simulink model "DAQ_DB_Test"  (Simulink 4.00)
settings: Solver=FixedStepDiscrete  StartTime=0.0  StopTime=inf  FixedStep=0.05  RelTol=1e-3
settings Model: LastModifiedBy=bsaunder

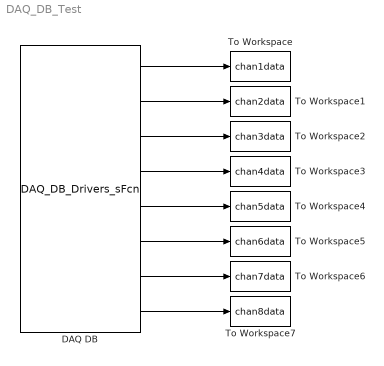
== system DAQ_DB_Test ==
  DAQ DB : S-Function  FunctionName=DAQ_DB_Drivers_sFcn  Parameters=Ts, (channels-1), gains, scanRate  PortCounts=[]  SFunctionModules=''  mask(DAQ_DB){channels=[1 2 3 4 5 6 7 8], gains=[1 1 1 1 1 1 1 1], scanRate=150, Ts=0.05}
      mask prompts: scanRate "Number of scans per sample time"; Ts "Sample time"
  To Workspace : ToWorkspace  VariableName=chan1data  SampleTime=-1  SaveFormat=Array
  To Workspace1 : ToWorkspace  VariableName=chan2data  SampleTime=-1  SaveFormat=Array
  To Workspace2 : ToWorkspace  VariableName=chan3data  SampleTime=-1  SaveFormat=Array
  To Workspace3 : ToWorkspace  VariableName=chan4data  SampleTime=-1  SaveFormat=Array
  To Workspace4 : ToWorkspace  VariableName=chan5data  SampleTime=-1  SaveFormat=Array
  To Workspace5 : ToWorkspace  VariableName=chan6data  SampleTime=-1  SaveFormat=Array
  To Workspace6 : ToWorkspace  VariableName=chan7data  SampleTime=-1  SaveFormat=Array
  To Workspace7 : ToWorkspace  VariableName=chan8data  SampleTime=-1  SaveFormat=Array
  wires:
  DAQ DB/1 -> To Workspace/1
  DAQ DB/2 -> To Workspace1/1
  DAQ DB/3 -> To Workspace2/1
  DAQ DB/4 -> To Workspace3/1
  DAQ DB/5 -> To Workspace4/1
  DAQ DB/6 -> To Workspace5/1
  DAQ DB/7 -> To Workspace6/1
  DAQ DB/8 -> To Workspace7/1
